simulink model "accFeedbackModel"  (R2014a)
settings: Solver=ode45  StartTime=0.0  StopTime=10.0  RelTol=1e-3
values from neighbouring files (symbols this model uses):
  Ki = PI.Ki    [accFeedbackOpt.m]    (also in gyrFeedbackOpt.m; notchFeedbackOpt.m; rawFeedbackOpt.m; strainFeedbackOpt.m)
  Kp = PI.Kp    [accFeedbackOpt.m]    (also in gyrFeedbackOpt.m; notchFeedbackOpt.m; rawFeedbackOpt.m; strainFeedbackOpt.m)
  Kq = -0.021    [accFeedback.m]    (also in accFeedbackOpt.m = Kq.d; gyrFeedbackOpt.m = Kq.d; gyroFeedback.m = -0.022; notchFeedbackOpt.m = Kq.d)
  KSa = -0.16    [accFeedbackOpt.m]
libraries: simulink x1
settings Model: CovSFcnEnable=on  Creator=anatole  LastModifiedBy=s220385
settings OptimizationCC: SimCompilerOptimization=off
settings DebuggingCC: MergeDetectMultiDrivingBlocksExec=error  SolverPrmCheckMsg=none  FrameProcessingCompatibilityMsg=error
settings RTWCC: RTWCompilerOptimization=off

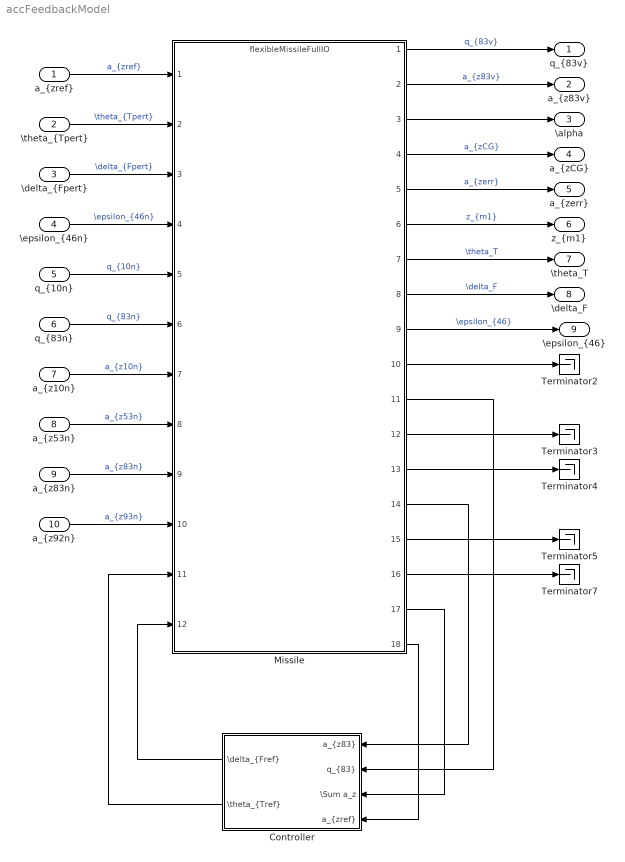
== system accFeedbackModel ==
  "a_{zref}" : Inport
  "\\theta_{Tpert}" : Inport  Port=2
  "\\delta_{Fpert}" : Inport  Port=3
  "\\epsilon_{46n}" : Inport  Port=4
  "q_{10n}" : Inport  Port=5
  "q_{83n}" : Inport  Port=6
  "a_{z10n}" : Inport  Port=7
  "a_{z53n}" : Inport  Port=8
  "a_{z83n}" : Inport  Port=9
  "a_{z92n}" : Inport  Port=10
  Controller : Subsystem
  Missile : ModelReference  ModelNameDialog=flexibleMissileFullIO.slx  SimulationMode=Normal  ModelReferenceVersion=1.74  CopyOfModelName=flexibleMissileFullIO.slx  DefaultDataLogging=on
  Terminator{2..5,7} (5 alike) : Terminator
  "q_{83v}" : Outport
  "a_{z83v}" : Outport  Port=2
  \alpha : Outport  Port=3
  "a_{zCG}" : Outport  Port=4
  "a_{zerr}" : Outport  Port=5
  "z_{m1}" : Outport  Port=6
  \theta_T : Outport  Port=7
  \delta_F : Outport  Port=8
  "\\epsilon_{46}" : Outport  Port=9
  wires:
  Controller/1("\\delta_{Fref}") -> Missile/12
  Controller/2("\\theta_{Tref}") -> Missile/11
  Missile/14 -> Controller/1("a_{z83}")
  Missile/11 -> Controller/2("q_{83}")
  Missile/18 -> Controller/4("a_{zref}")
  Missile/10 -> Terminator2/1
  Missile/12 -> Terminator3/1
  Missile/13 -> Terminator4/1
  Missile/15 -> Terminator5/1
  Missile/16 -> Terminator7/1
  Missile/17 -> Controller/3(\Sum a_z)
  "\\epsilon_{46n}"/1 -> Missile/4  "\\epsilon_{46n}"
  "q_{83n}"/1 -> Missile/6  "q_{83n}"
  "a_{z10n}"/1 -> Missile/7  "a_{z10n}"
  "a_{zref}"/1 -> Missile/1  "a_{zref}"
  "\\theta_{Tpert}"/1 -> Missile/2  "\\theta_{Tpert}"
  "a_{z92n}"/1 -> Missile/10  "a_{z93n}"
  "\\delta_{Fpert}"/1 -> Missile/3  "\\delta_{Fpert}"
  "q_{10n}"/1 -> Missile/5  "q_{10n}"
  "a_{z83n}"/1 -> Missile/9  "a_{z83n}"
  "a_{z53n}"/1 -> Missile/8  "a_{z53n}"
  Missile/1 -> "q_{83v}"/1  "q_{83v}"
  Missile/2 -> "a_{z83v}"/1  "a_{z83v}"
  Missile/6 -> "z_{m1}"/1  "z_{m1}"
  Missile/3 -> \alpha/1
  Missile/4 -> "a_{zCG}"/1  "a_{zCG}"
  Missile/5 -> "a_{zerr}"/1  "a_{zerr}"
  Missile/8 -> \delta_F/1  "\\delta_F"
  Missile/7 -> \theta_T/1  "\\theta_T"
  Missile/9 -> "\\epsilon_{46}"/1  "\\epsilon_{46}"

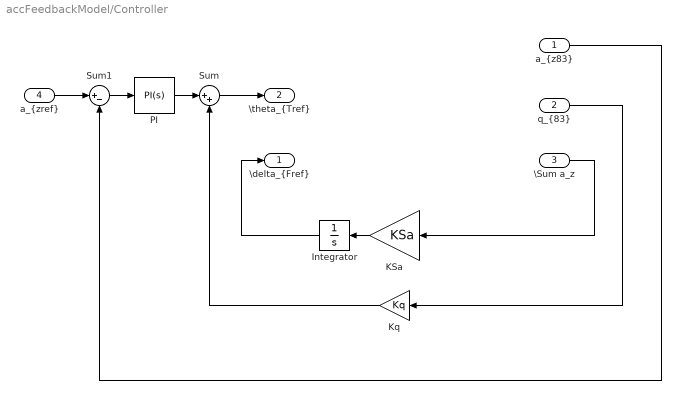
== system accFeedbackModel/Controller ==
  "a_{z83}" : Inport
  "q_{83}" : Inport  Port=2
  \Sum a_z : Inport  Port=3
  "a_{zref}" : Inport  Port=4
  Integrator : Integrator
  KSa : Gain  Gain=KSa
  Kq : Gain  Gain=Kq
  PI : simulink/Continuous/PID Controller  Controller=PI  TimeDomain=Continuous-time  SampleTime=-1  IntegratorMethod=Forward Euler  FilterMethod=Forward Euler  Form=Parallel  P=Kp  I=Ki  D=0  N=100  InitialConditionSource=internal  InitialConditionForIntegrator=0  InitialConditionForFilter=0  ExternalReset=none  LimitOutput=off  UpperSaturationLimit=inf  LowerSaturationLimit=-inf  LinearizeAsGain=on  AntiWindupMode=none  Kb=1  TrackingMode=off  Kt=1  PParamMin=[]  PParamMax=[]  IParamMin=[]  IParamMax=[]  DParamMin=[]  DParamMax=[]  NParamMin=[]  NParamMax=[]  KbParamMin=[]  KbParamMax=[]  KtParamMin=[]  KtParamMax=[]  POutMin=[]  POutMax=[]  IOutMin=[]  IOutMax=[]  DOutMin=[]  DOutMax=[]  NOutMin=[]  NOutMax=[]  KbOutMin=[]  KbOutMax=[]  KtOutMin=[]  KtOutMax=[]  IntegratorOutMin=[]  IntegratorOutMax=[]  FilterOutMin=[]  FilterOutMax=[]  SumOutMin=[]  SumOutMax=[]  SumI1OutMin=[]  SumI1OutMax=[]  SumI2OutMin=[]  SumI2OutMax=[]  SumI3OutMin=[]  SumI3OutMax=[]  SumDOutMin=[]  SumDOutMax=[]  SaturationOutMin=[]  SaturationOutMax=[]  IntegratorContinuousStateAttributes=''  IntegratorStateMustResolveToSignalObject=off  IntegratorRTWStateStorageClass=Auto  FilterContinuousStateAttributes=''  FilterStateMustResolveToSignalObject=off  FilterRTWStateStorageClass=Auto
  Sum : Sum  Inputs=|++
  Sum1 : Sum  Inputs=|+-
  "\\delta_{Fref}" : Outport
  "\\theta_{Tref}" : Outport  Port=2
  wires:
  KSa/1 -> Integrator/1
  Sum/1 -> "\\theta_{Tref}"/1
  \Sum a_z/1 -> KSa/1
  "q_{83}"/1 -> Kq/1
  Kq/1 -> Sum/2
  PI/1 -> Sum/1
  Sum1/1 -> PI/1
  "a_{zref}"/1 -> Sum1/1
  "a_{z83}"/1 -> Sum1/2
  Integrator/1 -> "\\delta_{Fref}"/1
